simulink library "headingSetpointwithWarpingCalculation_cl"  (R2018a)
settings: Solver=VariableStepAuto  StartTime=0.0  StopTime=10.0  RelTol=1e-3
libraries: flatlandHeading_ul x1, offsetLeadDistance_ul x1, pathPositionWithWarping_ul x1, pathProjectionWithWarping_ul x1
settings Model: Creator=mcobb  LastModifiedBy=mcobb

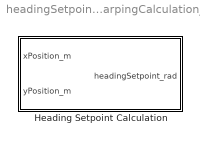
== system headingSetpointwithWarpingCalculation_cl ==
  Heading Setpoint Calculation : Subsystem

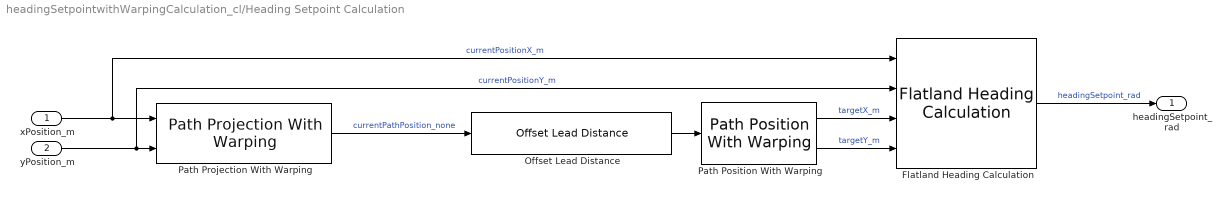
== system headingSetpointwithWarpingCalculation_cl/Heading Setpoint Calculation ==
  xPosition_m : Inport
  yPosition_m : Inport  Port=2
  Flatland Heading Calculation : flatlandHeading_ul/Flatland Heading Calculation
  Offset Lead Distance : offsetLeadDistance_ul/Offset Lead Distance
  Path Position With Warping : pathPositionWithWarping_ul/Path Position With Warping
  Path Projection With Warping : pathProjectionWithWarping_ul/Path Projection With Warping
  headingSetpoint_rad : Outport
  wires:
  Offset Lead Distance/1 -> Path Position With Warping/1
  Flatland Heading Calculation/1 -> headingSetpoint_rad/1  "headingSetpoint_rad"
  Path Projection With Warping/1 -> Offset Lead Distance/1  "currentPathPosition_none"
  Path Position With Warping/1 -> Flatland Heading Calculation/3  "targetX_m"
  Path Position With Warping/2 -> Flatland Heading Calculation/4  "targetY_m"
  xPosition_m/1 -> Path Projection With Warping/1, Flatland Heading Calculation/1  "currentPositionX_m"
  yPosition_m/1 -> Path Projection With Warping/2, Flatland Heading Calculation/2  "currentPositionY_m"
